simulink model "simlink13"  (R2017b)
settings: Solver=VariableStepAuto  StartTime=0.0  StopTime=10  RelTol=1e-3
settings Model: Creator=Administrator  LastModifiedBy=Administrator

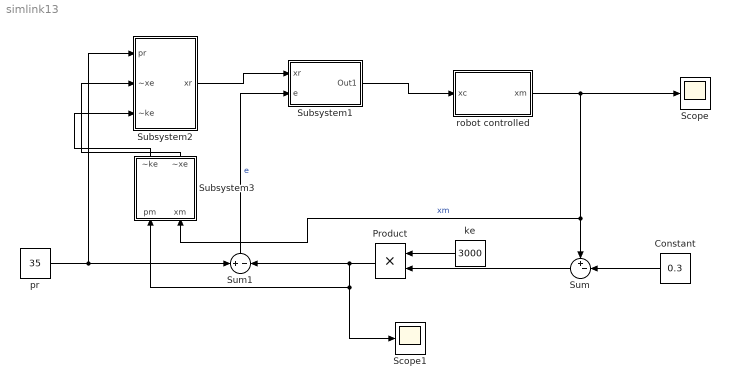
== system simlink13 ==
  Constant : Constant  Value=0.3
  Product : Product
  Scope : Scope
  Scope1 : Scope
  Subsystem1 : Subsystem
  Subsystem2 : Subsystem
  Subsystem3 : Subsystem
  Sum : Sum  Inputs=+-|
  Sum1 : Sum  Inputs=+|-
  ke : Constant  Value=3000
  pr : Constant  Value=35
  robot controlled : Subsystem
  wires:
  Subsystem3/1(~ke) -> Subsystem2/3(~ke)
  pr/1 -> Subsystem2/1(pr), Sum1/1
  Subsystem3/2(~xe) -> Subsystem2/2(~xe)
  Sum1/1 -> Subsystem1/2(e)  "e"
  Subsystem2/1(xr) -> Subsystem1/1(xr)
  Subsystem1/1(Out1) -> robot controlled/1(xc)
  Product/1 -> Scope1/1, Subsystem3/1(pm), Sum1/2
  Sum/1 -> Product/2
  robot controlled/1("xm ") -> Subsystem3/2(xm), Sum/1, Scope/1  "xm"
  ke/1 -> Product/1
  Constant/1 -> Sum/2

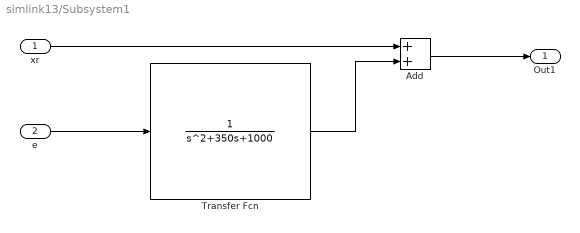
== system simlink13/Subsystem1 ==
  xr : Inport
  e : Inport  Port=2
  Add : Sum
  Transfer Fcn : TransferFcn  Denominator=[1 350 1000]
  Out1 : Outport
  wires:
  e/1 -> Transfer Fcn/1
  xr/1 -> Add/1
  Transfer Fcn/1 -> Add/2
  Add/1 -> Out1/1

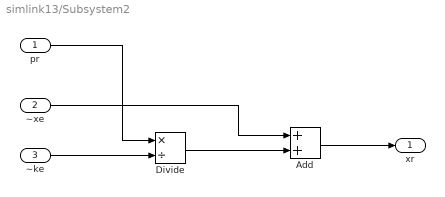
== system simlink13/Subsystem2 ==
  pr : Inport
  ~xe : Inport  Port=2
  ~ke : Inport  Port=3
  Add : Sum
  Divide : Product  Inputs=*/
  xr : Outport
  wires:
  pr/1 -> Divide/1
  ~ke/1 -> Divide/2
  ~xe/1 -> Add/1
  Divide/1 -> Add/2
  Add/1 -> xr/1

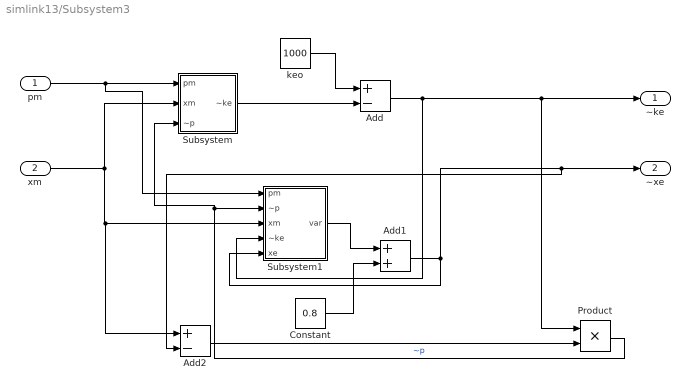
== system simlink13/Subsystem3 ==
  pm : Inport
  xm : Inport  Port=2
  Add : Sum  Inputs=+-
  Add1 : Sum
  Add2 : Sum  Inputs=+-
  Constant : Constant  Value=0.8
  Product : Product
  Subsystem : Subsystem
  Subsystem1 : Subsystem
  keo : Constant  Value=1000
  ~ke : Outport
  ~xe : Outport  Port=2
  wires:
  pm/1 -> Subsystem1/1(pm), Subsystem/1(pm)
  xm/1 -> Subsystem/2(xm), Add2/1, Subsystem1/3(xm)
  Add/1 -> Subsystem1/4(~ke), Product/1, ~ke/1
  Subsystem/1(~ke) -> Add/2
  Subsystem1/1(var) -> Add1/1
  Add1/1 -> Subsystem1/5("xe "), Add2/2, ~xe/1
  Add2/1 -> Product/2
  Product/1 -> Subsystem/3(~p), Subsystem1/2(~p)  "~p"
  keo/1 -> Add/1
  Constant/1 -> Add1/2

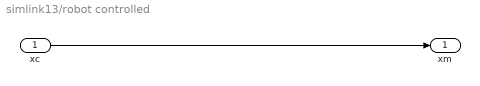
== system simlink13/robot controlled ==
  xc : Inport
  "xm " : Outport
  wires:
  xc/1 -> "xm "/1

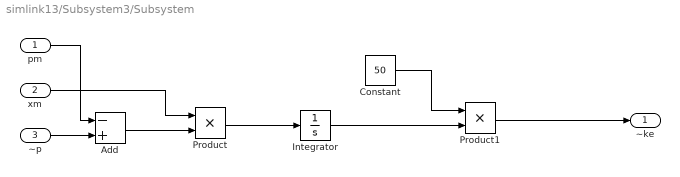
== system simlink13/Subsystem3/Subsystem ==
  pm : Inport
  xm : Inport  Port=2
  ~p : Inport  Port=3
  Add : Sum  Inputs=-+
  Constant : Constant  Value=50
  Integrator : Integrator
  Product : Product
  Product1 : Product
  ~ke : Outport
  wires:
  ~p/1 -> Add/2
  pm/1 -> Add/1
  xm/1 -> Product/1
  Add/1 -> Product/2
  Product/1 -> Integrator/1
  Integrator/1 -> Product1/2
  Product1/1 -> ~ke/1
  Constant/1 -> Product1/1

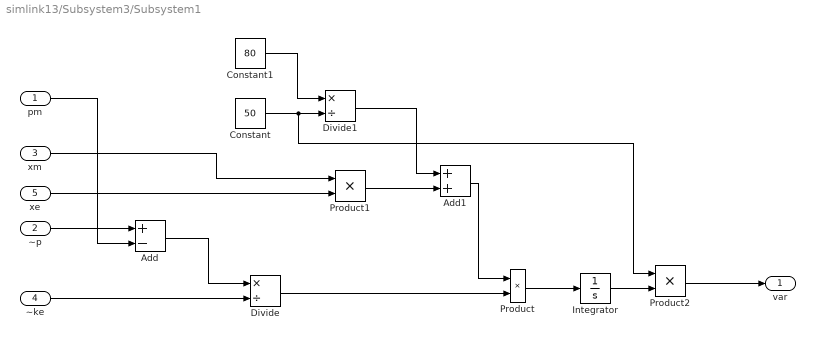
== system simlink13/Subsystem3/Subsystem1 ==
  pm : Inport
  ~p : Inport  Port=2
  xm : Inport  Port=3
  ~ke : Inport  Port=4
  "xe " : Inport  Port=5
  Add : Sum  Inputs=+-
  Add1 : Sum
  Constant : Constant  Value=50
  Constant1 : Constant  Value=80
  Divide : Product  Inputs=*/
  Divide1 : Product  Inputs=*/
  Integrator : Integrator
  Product : Product
  Product1 : Product
  Product2 : Product
  var : Outport
  wires:
  pm/1 -> Add/2
  ~p/1 -> Add/1
  Add/1 -> Divide/1
  ~ke/1 -> Divide/2
  Divide/1 -> Product/2
  xm/1 -> Product1/1
  Divide1/1 -> Add1/1
  Product1/1 -> Add1/2
  Add1/1 -> Product/1
  Integrator/1 -> Product2/2
  Product2/1 -> var/1
  "xe "/1 -> Product1/2
  Product/1 -> Integrator/1
  Constant1/1 -> Divide1/1
  Constant/1 -> Product2/1, Divide1/2
